simulink model "regulator_pouzeI"  (Simulink 7.6)
settings: Solver=ode45  StartTime=0.0  StopTime=20  RelTol=1e-3
settings Model: Creator=kaskaj  LastModifiedBy=kaskaj

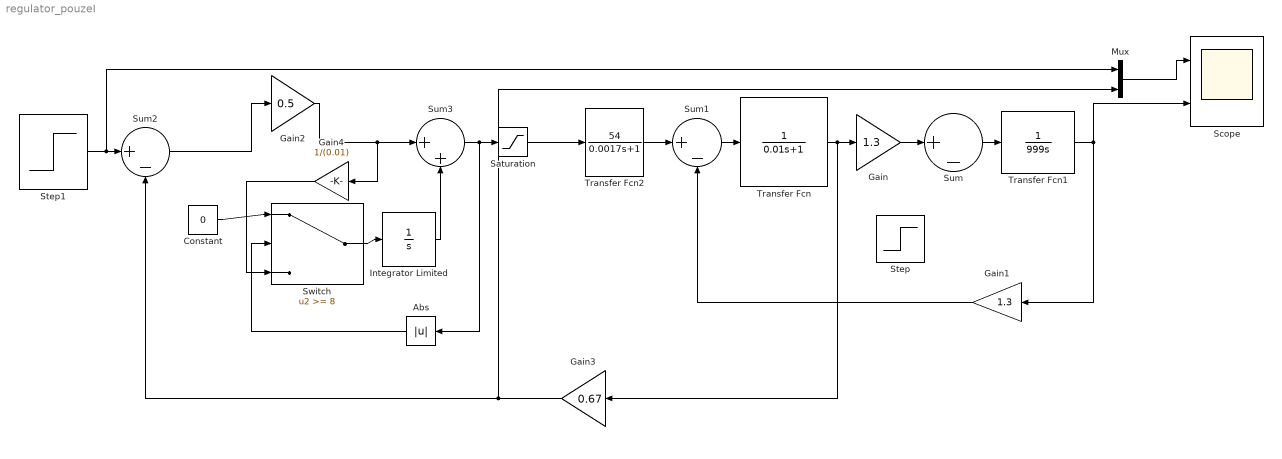
== system regulator_pouzeI ==
  Abs : Abs
  Constant : Constant  Value=0
  Gain : Gain  Gain=1.3
  Gain1 : Gain  Gain=1.3
  Gain2 : Gain  Gain=0.5
  Gain3 : Gain  Gain=0.67
  Gain4 : Gain  Gain=1/(0.01)
  Integrator Limited : Integrator  LimitOutput=on  UpperSaturationLimit=8  LowerSaturationLimit=-8
  Mux : Mux  Inputs=2
  Saturation : Saturate  UpperLimit=8  LowerLimit=-8
  Scope : Scope  NumInputPorts=2
      settings: YMin=-5~-5  YMax=5~5
  Step : Step  Time=5  After=5  SampleTime=0
  Step1 : Step  Time=2  After=5
  Sum : Sum  Inputs=|+-
  Sum1 : Sum  Inputs=|+-
  Sum2 : Sum  Inputs=|+-
  Sum3 : Sum  Inputs=|++
  Switch : Switch  Threshold=8
  Transfer Fcn : TransferFcn  Denominator=[0.01 1]
  Transfer Fcn1 : TransferFcn  Denominator=[999 0]
  Transfer Fcn2 : TransferFcn  Numerator=[54]  Denominator=[0.0017 1]
  wires:
  Transfer Fcn/1 -> Gain/1, Gain3/1
  Gain/1 -> Sum/1
  Sum/1 -> Transfer Fcn1/1
  Sum1/1 -> Transfer Fcn/1
  Transfer Fcn1/1 -> Gain1/1, Scope/2
  Gain1/1 -> Sum1/2
  Transfer Fcn2/1 -> Sum1/1
  Sum2/1 -> Gain2/1
  Gain2/1 -> Sum3/1, Gain4/1
  Switch/1 -> Integrator Limited/1
  Integrator Limited/1 -> Sum3/2
  Sum3/1 -> Abs/1, Saturation/1
  Saturation/1 -> Transfer Fcn2/1
  Gain3/1 -> Sum2/2, Mux/2
  Step1/1 -> Sum2/1, Mux/1
  Mux/1 -> Scope/1
  Gain4/1 -> Switch/3
  Constant/1 -> Switch/1
  Abs/1 -> Switch/2
